simulink model "FeedbackLinearizationModel"  (R2021a)
settings: Solver=VariableStepAuto  StartTime=0.0  StopTime=10.0  RelTol=1e-3
settings Model: Creator=Ali Rizvi  LastModifiedBy=Ali Rizvi

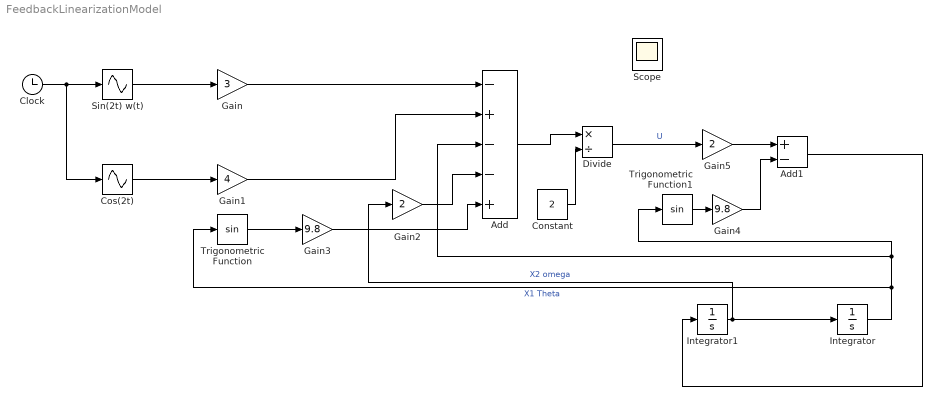
== system FeedbackLinearizationModel ==
  Add : Sum  Inputs=-+--+
  Add1 : Sum  Inputs=+-
  Clock : Clock
  Constant : Constant  Value=2
  "Cos(2t) " : Sin  TimeSource=Use external signal  Frequency=2  Phase=90  SampleTime=0
  Divide : Product  Inputs=*/
  Gain : Gain  Gain=3
  Gain1 : Gain  Gain=4
  Gain2 : Gain  Gain=2
  Gain3 : Gain  Gain=9.8
  Gain4 : Gain  Gain=9.8
  Gain5 : Gain  Gain=2
  Integrator : Integrator
  Integrator1 : Integrator
  Scope : Scope
  Sin(2t) w(t) : Sin  TimeSource=Use external signal  Frequency=2  SampleTime=0
  Trigonometric Function : Trigonometry
  Trigonometric Function1 : Trigonometry
  wires:
  Clock/1 -> "Cos(2t) "/1, Sin(2t) w(t)/1
  Sin(2t) w(t)/1 -> Gain/1
  Gain/1 -> Add/1
  "Cos(2t) "/1 -> Gain1/1
  Gain1/1 -> Add/2
  Integrator/1 -> Trigonometric Function1/1, Add/3, Trigonometric Function/1  "X1 Theta"
  Integrator1/1 -> Gain2/1, Integrator/1  "X2 omega"
  Gain2/1 -> Add/4
  Gain3/1 -> Add/5
  Trigonometric Function/1 -> Gain3/1
  Add/1 -> Divide/1
  Divide/1 -> Gain5/1  "U"
  Constant/1 -> Divide/2
  Gain5/1 -> Add1/1
  Trigonometric Function1/1 -> Gain4/1
  Gain4/1 -> Add1/2
  Add1/1 -> Integrator1/1
